simulink model "Wind_Testrig_org"  (Simulink 10.0)
settings: Solver=ode23t  StartTime=0.0  StopTime=400  RelTol=1e-5  EnableMultiTasking=on
PostLoadFcn:
  | warning off Simulink:blocks:MatchingGotoNotFound
  | warning off Simulink:blocks:MatchingFromNotFound
  | warning off Simulink:Engine:UsingDefaultMaxStepSize
undefined symbols (not defined in the file): Actuator_Lookup, radps2rpm, sigbuilder_block
libraries: sm_lib x3, Wind_Lib x1, Blades_Lib x1, Pitch_Controller_Lib x1, Pitch_System_Lib x1, Hub_Axis_Lib x1, nesl_utility x1
Description:
  | Copyright 2009-2017 The MathWorks, Inc. MathWorks, Inc.
settings Model: Creator=smiller  LastModifiedBy=bhisma
settings DataIOCC: LimitDataPoints=on
settings OptimizationCC: ExpressionDepthLimit=2147483647
settings DebuggingCC: SolverPrmCheckMsg=warning  FcnCallInpInsideContextMsg=warning  AllowSymbolicDim=off  StateNameClashWarn=warning
settings SFSimCC: SimParseCustomCode=off
settings GRTTargetCC: GeneratePreprocessorConditionals=Disable all
settings ConfigComp: CovExternalEMLEnable=off  CovSFcnEnable=off
settings SimscapeCC: SimscapeNormalizeSystem=off  SimscapeNominalValues="[{\"value\":\"10\",\"unit\":\"V\"},{\"value\":\"1\",\"unit\":\"A\"},{\"value\":\"10\",\"unit\":\"N*m\"},{\"value\":\"10\",\"unit\":\"bar\"},{\"value\":\"100\",\"unit\":\"kJ/kg\"},{\"value\":\"1\",\"unit\":\"kW\"},{\"value\":\"300\",\"unit\":\"K\"},{\"value\":\"100\",\"unit\":\"cm^3/s\"},{\"value\":\"1\",\"unit\":\"kN\"},{\"value\":\"1\",\"unit\":\"g/cm^3\"},{\"value\":\"1\",\"unit\":\"l\"},{\"value\":\"1\",\"unit\":\"cm^2\"},{\"value\":\"60\",\"unit\":\"Hz\"}]"
settings SimMechanicsCC: AnimationDelay=0  LastVizWinPosition=[420 528 560 420]  CamPosition=[-56.1901;-28.4673;10.4676;]  CamTarget=[1.18056;0.101824;-0.229298;]  CamUpVector=[0.179671;0.00751397;0.983698;]  CamHeight=4.38469  VisBackgroundColor=[0.9;0.9;0.95;]  DefaultBodyColor=[1;0;0;]
settings ConfigurationSet: Description=SimMechanics 2G
settings ExplorerConfigSet: InternalSimMechanicsExplorerSettings="<ExplorerConfiguration><canonicalview>default</canonicalview><TilePanel><TileInfo><Tiles Columns=\"1\" Count=\"1\" Rows=\"1\"><Column Left=\"2\" Weight=\"1\"/><Column Left=\"651\"/><Row Top=\"2\" Weight=\"1\"/><Row Top=\"510\"/><Tile Height=\"1\" Width=\"1\" X=\"0\" Y=\"0\"/></Tiles></TileInfo><SceneInfo><SceneViewer><BGColor><R>0.80000001192092896</R><G>1</G><B>1</B></BGColor><Camera><Position><X>-18.34444732617348</X><Y>-79.064377059046635</Y><Z>61.050217652840232</Z></Position><Center><X>-9.635435577615457</X><Y>1.1439116155005564</Y><Z>1.7946145717997837</Z></Center><Up><X>-0.063772345088641574</X><Y>0.59746516561897667</Y><Z>0.79935502992962004</Z></Up><Left>-34.087521171569826</Left><Right>34.087521171569826</Right><Bottom>-3.1111695885658266</Bottom><Top>3.1111695885658266</Top></Camera></SceneViewer></SceneInfo></TilePanel></ExplorerConfiguration>"

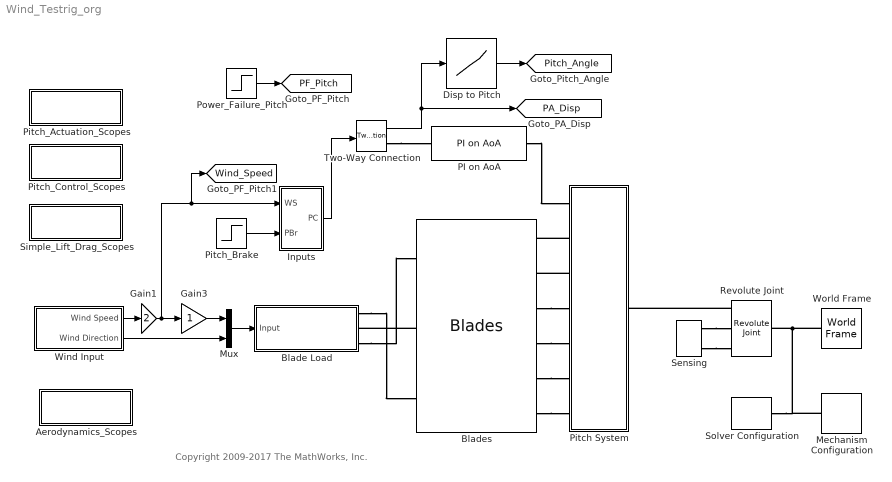
== system Wind_Testrig_org ==
  note: Copyright 2009-2017 The MathWorks, Inc.
  Aerodynamics_Scopes : Subsystem  AncestorBlock=Wind_Lib/Simple_Lift_Drag_Scopes
  Blade Load : Subsystem  BlockChoice=Segments
      settings: AttributesFormatString=%<BlockChoice>  TemplateBlock=Wind_Lib/Blade Load  MemberBlocks=Lift and Drag,Lift and Drag Simscape,Segments,Torque
      mask Display: disp(' ');
  Blades : Blades_Lib/Blades  SystemSampleTime=-1
  Disp to Pitch : Lookup  InputValues=Actuator_Lookup.extension  Table=Actuator_Lookup.angle
  Gain1 : Gain  Gain=2
  Gain3 : Gain
  Inputs : Subsystem
  Mechanism Configuration : sm_lib/Utilities/Mechanism Configuration  UniformGravity=Constant  GravityVector=[0 0 -9.81]  GravityUnits=m/s^2  LinearizationDelta=0.001
  Mux : Mux  Inputs=2
  PI on AoA : Pitch_Controller_Lib/PI on AoA  SystemSampleTime=-1
  Pitch System : Subsystem  BlockChoice=Ideal
      settings: AttributesFormatString=%<BlockChoice>  TemplateBlock=Pitch_System_Lib/Pitch System  MemberBlocks=Hydraulic,Ideal,Locked
      mask Display: disp(' ');
  Pitch_Actuation_Scopes : Subsystem
  Pitch_Brake : Step  After=0  SampleTime=0
  Pitch_Control_Scopes : Subsystem
  Power_Failure_Pitch : Step  Time=5  Before=24  After=24  SampleTime=0
  Revolute Joint : sm_lib/Joints/Revolute Joint  JointMode=Normal  SenseConstraintForce=off  SenseConstraintForceX=off  SenseConstraintForceY=off  SenseConstraintForceZ=off  SenseConstraintTorque=off  SenseConstraintTorqueX=off  SenseConstraintTorqueY=off  SenseConstraintTorqueZ=off  SenseTotalForce=off  SenseTotalForceX=off  SenseTotalForceY=off  SenseTotalForceZ=off  SenseTotalTorque=off  SenseTotalTorqueX=off  SenseTotalTorqueY=off  SenseTotalTorqueZ=off  CompositeWrenchDir=FollowerOnBase  CompositeWrenchFrame=BaseFrame  EquilibriumPosition=0  EquilibriumPositionUnits=deg  SpringStiffness=0  SpringStiffnessUnits=N*m/deg  DampingCoefficient=0  DampingCoefficientUnits=N*m/(deg/s)  TorqueActuationMode=NoTorque  MotionActuationMode=ComputedMotion  SensePosition=on  SenseVelocity=on  SenseAcceleration=off  SenseTorqueForce=off  SenseLowerLimitTorqueForce=off  SenseUpperLimitTorqueForce=off  LowerLimitSpecify=off  LowerLimitBound=-90  LowerLimitBoundUnits=deg  LowerLimitStiffness=1e4  LowerLimitStiffnessUnits=N*m/deg  LowerLimitDamping=10  LowerLimitDampingUnits=N*m/(deg/s)  LowerLimitTransitionRegionWidth=0.1  LowerLimitTransitionRegionWidthUnits=deg  UpperLimitSpecify=off  UpperLimitBound=90  UpperLimitBoundUnits=deg  UpperLimitStiffness=1e4  UpperLimitStiffnessUnits=N*m/deg  UpperLimitDamping=10  UpperLimitDampingUnits=N*m/(deg/s)  UpperLimitTransitionRegionWidth=0.1  UpperLimitTransitionRegionWidthUnits=deg  PositionTargetSpecify=on  PositionTargetPriority=High  PositionTargetValue=0  PositionTargetValueUnits=deg  VelocityTargetSpecify=off  VelocityTargetPriority=High  VelocityTargetValue=0  VelocityTargetValueUnits=deg/s
  Sensing : Hub_Axis_Lib/Rotate/Sensing
  Simple_Lift_Drag_Scopes : Subsystem  AncestorBlock=Wind_Lib/Simple_Lift_Drag_Scopes
  Solver Configuration : nesl_utility/Solver Configuration  PhysicalDomain=network_engine_domain  SubClassName=solver  LeftPortType=input  RightPortType=generic  Tones=[]  Harmonics=[]  SimulateNoise=off  Profile=off  UseLocalSampling=off  EnableSwitchedLinearOptims=on  FrequencyDomain=off  UseCCode=off  RelTol=0.001  AbsTol=1e-06  MinStep=1e-09  ToWorkspace=off  RevertToSquareIcSolve=off  NumHomotopyIterations=100  PhasorMode=off  PhasorModeNumHarmonics=1  DoDC=off  ResidualTolerance=1e-9  UseLocalSolver=off  LocalSolverChoice=NE_BACKWARD_EULER_ADVANCER  LocalSolverSampleTime=.001  DoFixedCost=off  MaxNonlinIter=3  MaxModeIter=2  LinearAlgebra=Sparse  EquationFormulation=NE_TIME_EF  DelaysMemoryBudget=1024  AutomaticFiltering=on  FilteringTimeConstant=0.001  PartitionStorageMethod=AS_NEEDED  PartitionMemoryBudget=1024  PartitionMethod=FAST
  Two-Way Connection : TwoWayConnection
  Wind Input : Subsystem  Tag=STV Subsys  LoadFcn=sigbuilder_block('load');  StartFcn=sigbuilder_block('start');  StopFcn=sigbuilder_block('stop');  ClipboardFcn=sigbuilder_block('clipboard');  mask(Sigbuilder block){tuvar=[0:10]}
      mask help: Sigbuilder GUI
      mask init:
      | if ~strcmp(get_param(bdroot(gcbh),'SimulationStatus'),'stopped') tuvar = sigbuilder_block('maskInit'); end
      settings: CopyFcn=sigbuilder_block('copy');  DeleteFcn=sigbuilder_block('delete');  ModelCloseFcn=sigbuilder_block('modelClose');  PreSaveFcn=sigbuilder_block('preSave');  PauseFcn=sigbuilder_block('pause')  ContinueFcn=sigbuilder_block('continue')  NameChangeFcn=sigbuilder_block('namechange');  OpenFcn=sigbuilder_block('open',[33 180 762 399.75 ]);  CloseFcn=sigbuilder_block('close');
      mask Display: plot(0, 0, 100, 100,[2, 2, 32, 32, 2], [68, 8, 8, 68, 68],[32, 2], [38, 38], [32, 19, 2],[53, 60, 44], [32, 17, 17, 2],[16, 16, 31, 31]);txt = getActiveGroup(gcbh);text(2, 100, txt,'verticalAlignment', 'top');
  World Frame : sm_lib/Frames and Transforms/World Frame
  tag scope: PA_Disp=global, PF_Pitch=global, Pitch_Angle=global, Wind_Speed=global
  wires:
  Disp to Pitch/1 -> [Pitch_Angle]
  Two-Way Connection/1 -> [PA_Disp], Disp to Pitch/1
  Power_Failure_Pitch/1 -> [PF_Pitch]
  Wind Input/1(Wind Speed) -> Gain1/1
  Wind Input/2(Wind Direction) -> Mux/2
  Mux/1 -> Blade Load/1(Input)
  Pitch_Brake/1 -> Inputs/2(PBr)
  Inputs/1(PC) -> Two-Way Connection/1
  Gain3/1 -> Mux/1
  Gain1/1 -> Gain3/1, Inputs/1(WS), [Wind_Speed]
  connections:
  Pitch System/LConn2 -- Blades/LConn1
  Blades/LConn5 -- Pitch System/LConn6
  Blades/LConn3 -- Pitch System/LConn4
  Pitch System/LConn3 -- Blades/LConn2
  Two-Way Connection/RConn1 -- PI on AoA/LConn1
  PI on AoA/RConn1 -- Pitch System/LConn1
  Blades/LConn4 -- Pitch System/LConn5
  Blades/LConn6 -- Pitch System/LConn7
  Blade Load/RConn1 -- Blades/RConn3
  Blades/RConn2 -- Blade Load/RConn2
  Blade Load/RConn3 -- Blades/RConn1
  Sensing/LConn1 -- Revolute Joint/RConn2
  Sensing/LConn2 -- Revolute Joint/RConn3
  Revolute Joint/RConn1 -- Pitch System/RConn1
  World Frame/RConn1 -- Mechanism Configuration/RConn1 -- Solver Configuration/RConn1 -- Revolute Joint/LConn1

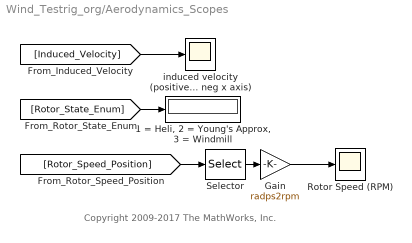
== system Wind_Testrig_org/Aerodynamics_Scopes ==
  note: Copyright 2009-2017 The MathWorks, Inc.
  "1 = Heli, 2 = Young's Approx, 3 = Windmill" : Display
  Gain : Gain  Gain=radps2rpm
  Rotor Speed (RPM) : Scope
  Selector : Selector  InputPortWidth=2  IndexOptions=Index vector (dialog)  Indices=[2]  OutputSizes=1
  induced velocity (positive in neg x axis) : Scope
  wires:
  [Rotor_State_Enum] -> "1 = Heli, 2 = Young's Approx, 3 = Windmill"/1
  [Induced_Velocity] -> induced velocity (positive in neg x axis)/1
  [Rotor_Speed_Position] -> Selector/1
  Selector/1 -> Gain/1
  Gain/1 -> Rotor Speed (RPM)/1

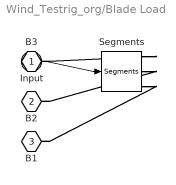
== system Wind_Testrig_org/Blade Load ==
  Input : Inport
  Segments : Wind_Lib/Segments  SystemSampleTime=-1
  B3 : PMIOPort  Side=Right
  B2 : PMIOPort  Port=2  Side=Right
  B1 : PMIOPort  Port=3  Side=Right
  wires:
  Input/1 -> Segments/1
  connections:
  Segments/RConn1 -- B3/RConn1
  Segments/RConn2 -- B2/RConn1
  Segments/RConn3 -- B1/RConn1

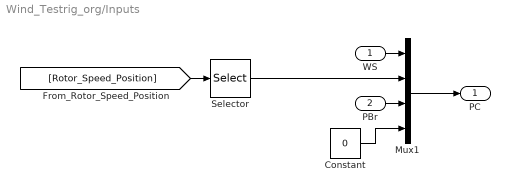
== system Wind_Testrig_org/Inputs ==
  WS : Inport
  PBr : Inport  Port=2
  Constant : Constant  Value=0
  Mux1 : Mux
  Selector : Selector  InputPortWidth=2  IndexOptions=Index vector (dialog)  Indices=[2]  OutputSizes=1
  PC : Outport
  wires:
  [Rotor_Speed_Position] -> Selector/1
  Selector/1 -> Mux1/2
  WS/1 -> Mux1/1
  Mux1/1 -> PC/1
  PBr/1 -> Mux1/3
  Constant/1 -> Mux1/4

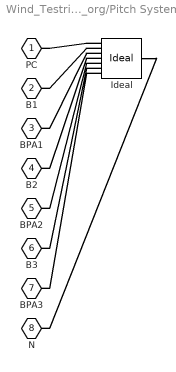
== system Wind_Testrig_org/Pitch System ==
  Ideal : Pitch_System_Lib/Ideal  SystemSampleTime=-1
  PC : PMIOPort  Side=Left
  B1 : PMIOPort  Port=2  Side=Left
  BPA1 : PMIOPort  Port=3  Side=Left
  B2 : PMIOPort  Port=4  Side=Left
  BPA2 : PMIOPort  Port=5  Side=Left
  B3 : PMIOPort  Port=6  Side=Left
  BPA3 : PMIOPort  Port=7  Side=Left
  N : PMIOPort  Port=8  Side=Right
  connections:
  Ideal/LConn1 -- PC/RConn1
  Ideal/LConn2 -- B1/RConn1
  Ideal/LConn3 -- BPA1/RConn1
  Ideal/LConn4 -- B2/RConn1
  Ideal/LConn5 -- BPA2/RConn1
  Ideal/LConn6 -- B3/RConn1
  Ideal/LConn7 -- BPA3/RConn1
  Ideal/RConn1 -- N/RConn1

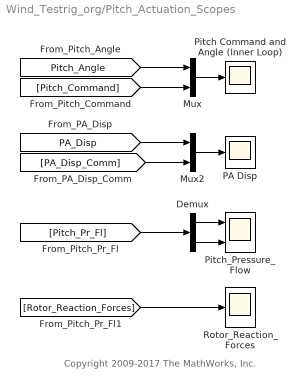
== system Wind_Testrig_org/Pitch_Actuation_Scopes ==
  note: Copyright 2009-2017 The MathWorks, Inc.
  Demux : Demux  Outputs=[2 1]
  Mux : Mux  Inputs=2
  Mux2 : Mux  Inputs=2
  PA Disp : Scope
  Pitch Command and Angle (Inner Loop) : Scope
  Pitch_Pressure_Flow : Scope  NumInputPorts=2
  Rotor_Reaction_Forces : Scope
  wires:
  [Pitch_Angle] -> Mux/1
  [Pitch_Command] -> Mux/2
  Mux/1 -> Pitch Command and Angle (Inner Loop)/1
  [PA_Disp] -> Mux2/1
  Mux2/1 -> PA Disp/1
  [PA_Disp_Comm] -> Mux2/2
  [Pitch_Pr_Fl] -> Demux/1
  Demux/1 -> Pitch_Pressure_Flow/1
  Demux/2 -> Pitch_Pressure_Flow/2
  [Rotor_Reaction_Forces] -> Rotor_Reaction_Forces/1

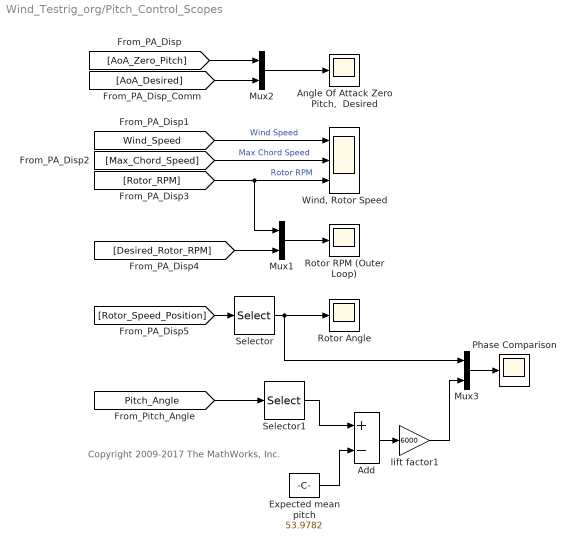
== system Wind_Testrig_org/Pitch_Control_Scopes ==
  note: Copyright 2009-2017 The MathWorks, Inc.
  Add : Sum  Inputs=+-
  "Angle Of Attack Zero Pitch,  Desired" : Scope
  Expected mean pitch : Constant  Value=53.9782
  Mux1 : Mux  Inputs=2
  Mux2 : Mux  Inputs=2
  Mux3 : Mux  Inputs=2
  Phase Comparison : Scope
  Rotor Angle : Scope
  Rotor RPM (Outer Loop) : Scope
  Selector : Selector  InputPortWidth=2  IndexOptions=Index vector (dialog)  Indices=[1]  OutputSizes=1
  Selector1 : Selector  InputPortWidth=3  IndexOptions=Index vector (dialog)  Indices=[1]  OutputSizes=1
  "Wind, Rotor Speed" : Scope  NumInputPorts=3
  lift factor1 : Gain  Gain=6000
  wires:
  [AoA_Desired] -> Mux2/2
  Mux2/1 -> "Angle Of Attack Zero Pitch,  Desired"/1
  [AoA_Zero_Pitch] -> Mux2/1
  [Wind_Speed] -> "Wind, Rotor Speed"/1  "Wind Speed"
  [Max_Chord_Speed] -> "Wind, Rotor Speed"/2  "Max Chord Speed"
  [Rotor_RPM] -> "Wind, Rotor Speed"/3, Mux1/1  "Rotor RPM"
  Mux1/1 -> Rotor RPM (Outer Loop)/1
  [Desired_Rotor_RPM] -> Mux1/2
  [Rotor_Speed_Position] -> Selector/1
  Selector/1 -> Rotor Angle/1, Mux3/1
  Mux3/1 -> Phase Comparison/1
  Expected mean pitch/1 -> Add/2
  [Pitch_Angle] -> Selector1/1
  Selector1/1 -> Add/1
  Add/1 -> lift factor1/1
  lift factor1/1 -> Mux3/2

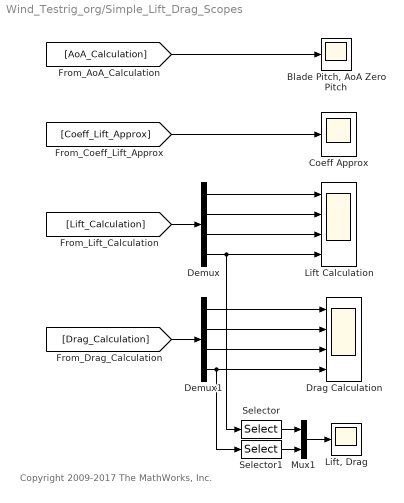
== system Wind_Testrig_org/Simple_Lift_Drag_Scopes ==
  note: Copyright 2009-2017 The MathWorks, Inc.
  "Blade Pitch, AoA Zero Pitch" : Scope
  Coeff Approx : Scope
  Demux : Demux  Outputs=[1 3 3 3]
  Demux1 : Demux  Outputs=[1 3 3 3]
  Drag Calculation : Scope  NumInputPorts=4
  Lift Calculation : Scope  NumInputPorts=4
  "Lift, Drag" : Scope
  Mux1 : Mux  Inputs=2
  Selector : Selector  InputPortWidth=3  IndexOptions=Index vector (dialog)  Indices=[1]  OutputSizes=1
  Selector1 : Selector  InputPortWidth=3  IndexOptions=Index vector (dialog)  Indices=[1 3]  OutputSizes=1
  wires:
  Demux1/4 -> Drag Calculation/4, Selector1/1
  Demux1/3 -> Drag Calculation/3
  Demux1/2 -> Drag Calculation/2
  Demux1/1 -> Drag Calculation/1
  [Drag_Calculation] -> Demux1/1
  [Coeff_Lift_Approx] -> Coeff Approx/1
  Demux/4 -> Lift Calculation/4, Selector/1
  Demux/3 -> Lift Calculation/3
  Demux/2 -> Lift Calculation/2
  Demux/1 -> Lift Calculation/1
  [Lift_Calculation] -> Demux/1
  Mux1/1 -> "Lift, Drag"/1
  [AoA_Calculation] -> "Blade Pitch, AoA Zero Pitch"/1
  Selector/1 -> Mux1/1
  Selector1/1 -> Mux1/2

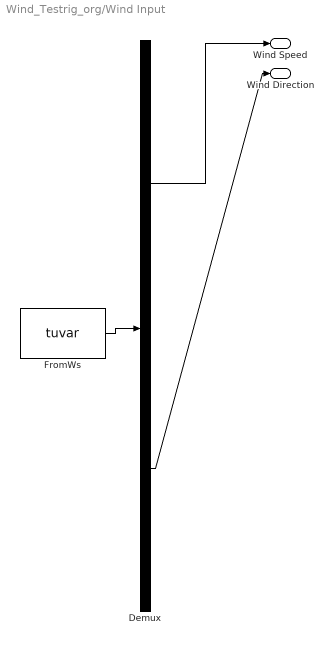
== system Wind_Testrig_org/Wind Input ==
  Demux : Demux  Tag=STV Demux  Outputs=2
  FromWs : FromWorkspace  Tag=STV FromWs  VariableName=tuvar  SampleTime=0  SigBuilderData=DataTag0  VnvData=DataTag1
      SigBuilderData=|
      | common.afterFinalStr = 'Extrapolate'
      | common.sampleTime = 0
      | dataSet(1).timeRange = [0 130]
      | dataSet(1).name = 'High Wind Speed'
      | dataSet(2).timeRange = [0 130]
      | dataSet(2).name = 'Constant Wind'
      | dataSet(3).timeRange = [0 130]
      | dataSet(3).name = 'Cut In'
      | sbobj.Groups(1).Name = 'High Wind Speed'
      | sbobj.Groups(1).Signals(1).Name = 'Wind Speed'
      | sbobj.Groups(1).Signals(1).XData = [0 10 10 25.1 28 91.8 100 130]
      | sbobj.Groups(1).Signals(1).YData = [10 10 9.9 9.9 5 5 8 10]
      | sbobj.Groups(1).Signals(2).Name = 'Wind Direction'
      | sbobj.Groups(1).Signals(2).XData = [0 1 1 11 11 21 21 31 31 130]
      | sbobj.Groups(1).Signals(2).YData = [0 0 4 4 0 0 -4 -4 0 0]
      | sbobj.Groups(2).Name = 'Constant Wind'
      | sbobj.Groups(2).Signals(1).Name = 'Wind Speed'
      | sbobj.Groups(2).Signals(1).XData = [0 10 130]
      | sbobj.Groups(2).Signals(1).YData = [10 10 10]
      | sbobj.Groups(2).Signals(2).Name = 'Wind Direction'
      | sbobj.Groups(2).Signals(2).XData = [0 1 1 11 11 21 21 31 31 130]
      | sbobj.Groups(2).Signals(2).YData = [0 0 4 4 0 0 -4 -4 0 0]
      | sbobj.Groups(3).Name = 'Cut In'
      | sbobj.Groups(3).Signals(1).Name = 'Wind Speed'
      | sbobj.Groups(3).Signals(1).XData = [0 25.1 28 91.8 100 121.8 130]
      | sbobj.Groups(3).Signals(1).YData = [4.5 8.7 7.85 9.65 8 10 10]
      | sbobj.Groups(3).Signals(2).Name = 'Wind Direction'
      | sbobj.Groups(3).Signals(2).XData = [0 1 1 11 11 21 21 31 31 130]
      | sbobj.Groups(3).Signals(2).YData = [0 0 4 4 0 0 -4 -4 0 0]
  Wind Speed : Outport  Tag=STV Outport
  Wind Direction : Outport  Tag=STV Outport  Port=2
  wires:
  Demux/2 -> Wind Direction/1
  Demux/1 -> Wind Speed/1
  FromWs/1 -> Demux/1
